simulink model "step_analysis_"  (R2023b)
settings: Solver=VariableStepAuto  StartTime=0.0  StopTime=10  RelTol=1e-3
values from neighbouring files (symbols this model uses):
  A_cond = A-B*inv(D)*C    [step_analysis.m]
  B_cond = B*inv(D)    [step_analysis.m]
  C = PID_ss.C    [step_analysis.m]
  D = PID_ss.D    [step_analysis.m]
  den = conv([tau1,1],[tau2,1])    [tentative.m]
  num = K    (= 0.0907194437342)    [tentative.m]
  t_step = t(ind)    [step_analysis.m]
  Ts_slk = 0.001    [step_analysis.m]
libraries: cstblocks x1
settings Model: Creator=alexz  LastModifiedBy=alexz

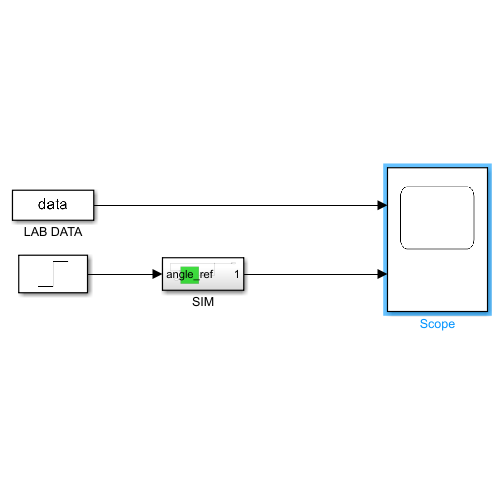
[thumbnail: Simulink's stored preview of the top-level diagram]
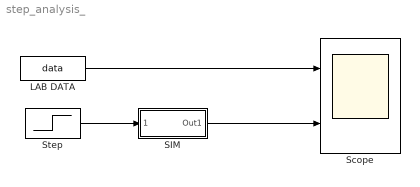
== system step_analysis_ ==
  LAB DATA : FromWorkspace  VariableName=data
  SIM : Subsystem
  Scope : Scope  NumInputPorts=2
  Step : Step  Time=t_step  After=0.0873  SampleTime=0
  wires:
  LAB DATA/1 -> Scope/1
  SIM/1(Out1) -> Scope/2
  Step/1 -> SIM/1(angle_ref)

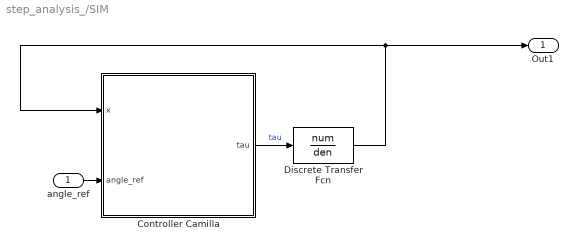
== system step_analysis_/SIM ==
  angle_ref : Inport
  Controller Camilla : Subsystem
  Discrete Transfer Fcn : DiscreteTransferFcn  Numerator=num  Denominator=den
  Out1 : Outport
  wires:
  Discrete Transfer Fcn/1 -> Out1/1, Controller Camilla/1(x)
  Controller Camilla/1(tau) -> Discrete Transfer Fcn/1  "tau"
  angle_ref/1 -> Controller Camilla/2(angle_ref)

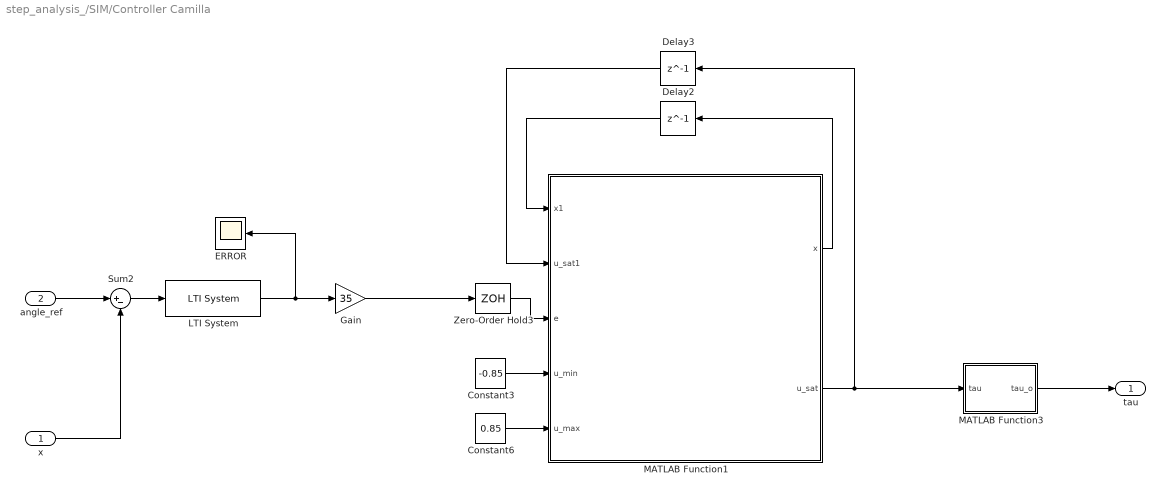
== system step_analysis_/SIM/Controller Camilla ==
  x : Inport
  angle_ref : Inport  Port=2
  Constant3 : Constant  Value=-0.85  SampleTime=Ts_slk
  Constant6 : Constant  Value=0.85  SampleTime=Ts_slk
  Delay2 : Delay  DelayLength=1  InitialCondition=zeros(2,1)  SampleTime=Ts_slk
  Delay3 : Delay  DelayLength=1  InitialCondition=0  SampleTime=Ts_slk
  ERROR : Scope
  Gain : Gain  Gain=35
  LTI System : cstblocks/LTI System  sys=filter_d  IC=[]  PadeOrder=0
  MATLAB Function1 : MATLAB Function  TreatAsAtomicUnit=on
  MATLAB Function3 : MATLAB Function  TreatAsAtomicUnit=on
  Sum2 : Sum  Inputs=|+-
  Zero-Order Hold3 : ZeroOrderHold  SampleTime=Ts_slk
  tau : Outport
  wires:
  angle_ref/1 -> Sum2/1
  MATLAB Function3/1(tau_o) -> tau/1
  Sum2/1 -> LTI System/1
  MATLAB Function1/2(u_sat) -> MATLAB Function3/1(tau), Delay3/1
  Gain/1 -> Zero-Order Hold3/1
  x/1 -> Sum2/2
  Constant6/1 -> MATLAB Function1/5(u_max)
  Zero-Order Hold3/1 -> MATLAB Function1/3(e)
  MATLAB Function1/1(x) -> Delay2/1
  Delay3/1 -> MATLAB Function1/2(u_sat1)
  Constant3/1 -> MATLAB Function1/4(u_min)
  Delay2/1 -> MATLAB Function1/1(x1)
  LTI System/1 -> ERROR/1, Gain/1

== matlab function step_analysis_/SIM/Controller Camilla/MATLAB Function1 ==
  data: x1 input; x output; u_sat1 input; e input; u_sat output; A_cond parameter; B_cond parameter; C parameter; D parameter; u_min input; u_max input
function [x,u_sat]= PID_controller(x1,u_sat1,e, A_cond, B_cond, C, D, u_min, u_max)%, on_off)
% if on_off == 0
%     x1 = zeros(2,1);
%     u_sat1 = 0;
% end
x       =   A_cond*x1 + B_cond*u_sat1;
u       =   C*x + D*e;
u_sat   =   max(u_min, min (u_max, u));  
end

== matlab function step_analysis_/SIM/Controller Camilla/MATLAB Function3 ==
  data: tau input; tau_o output
function tau_o=fcn(tau)
% Inputs:   tau    (torque 1x1)         
%
% Outputs:  tau_o  (torque 3x1)

% States in input
tau_1     =       tau(1,1);     %  roll torque

% States in output
tau_o =       tau_1;
